simulink model "linearFB"  (R2023a)
settings: Solver=VariableStepAuto  StartTime=0.0  StopTime=60  RelTol=1e-3
values from neighbouring files (symbols this model uses):
  eps_0 = [.2; -.5; .3]    [as5.m]
  eps_c = [-.2; -.4; .2]    [as5.m]
  eta_c = sqrt(1- eps_c'*eps_c)    [as5.m]
  I = [1200 0 0; 0 2000 0; 0 0 2800]    [as5.m]
  k_d = I * eye(3) * 2 * zeta * omega_n    [as5.m]
  k_p = I * eye(3) * 2 * omega_n^2    [as5.m]
  omega_0 = [.1; -.05; .05]    [as5.m]
settings Model: Creator=renob  LastModifiedBy=Josh2

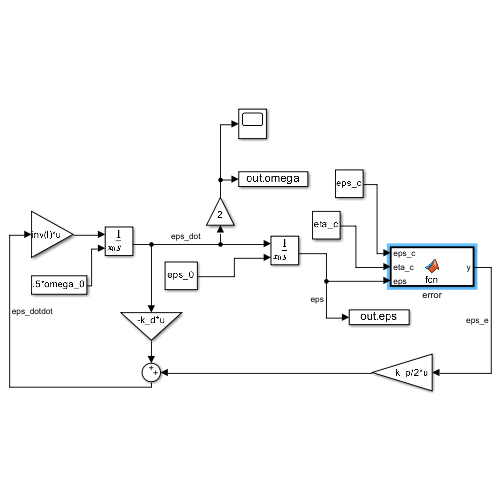
[thumbnail: Simulink's stored preview of the top-level diagram]
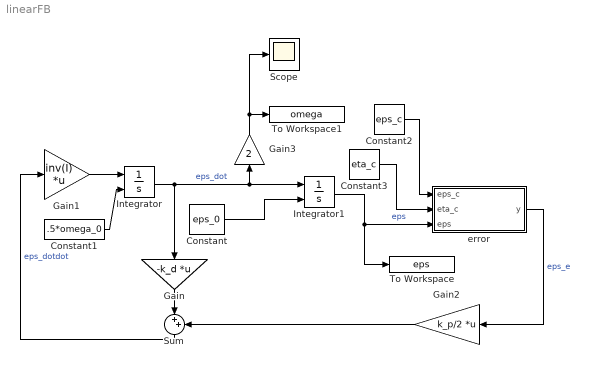
== system linearFB ==
  Constant : Constant  Value=eps_0
  Constant1 : Constant  Value=.5*omega_0
  Constant2 : Constant  Value=eps_c
  Constant3 : Constant  Value=eta_c
  Gain : Gain  Gain=-k_d  Multiplication=Matrix(K*u)
  Gain1 : Gain  Gain=inv(I)  Multiplication=Matrix(K*u)
  Gain2 : Gain  Gain=k_p/2  Multiplication=Matrix(K*u)
  Gain3 : Gain  Gain=2
  Integrator : Integrator  InitialConditionSource=external  InitialCondition=.5*omega_0
  Integrator1 : Integrator  InitialConditionSource=external
  Scope : Scope
  Sum : Sum  Inputs=|++
  To Workspace : ToWorkspace  VariableName=eps  SampleTime=-1
      settings: Save2DSignal=2-D array (concatenate along first dimension)
  To Workspace1 : ToWorkspace  VariableName=omega  SampleTime=-1
      settings: Save2DSignal=2-D array (concatenate along first dimension)
  error : MATLAB Function  TreatAsAtomicUnit=on
  wires:
  Integrator/1 -> Gain/1, Gain3/1, Integrator1/1  "eps_dot"
  Gain1/1 -> Integrator/1
  Integrator1/1 -> To Workspace/1, error/3(eps)  "eps"
  Gain/1 -> Sum/1
  Sum/1 -> Gain1/1  "eps_dotdot"
  Gain2/1 -> Sum/2
  Constant/1 -> Integrator1/2
  Constant1/1 -> Integrator/2
  Gain3/1 -> Scope/1, To Workspace1/1
  error/1(y) -> Gain2/1  "eps_e"
  Constant3/1 -> error/2(eta_c)
  Constant2/1 -> error/1(eps_c)

== matlab function linearFB/error ==
  data: eps_c input; eta_c input; eps input; y output
function y = fcn(eps_c, eta_c, eps)
eta = sqrt(1-eps'*eps);

q_e = quatmultiply(quatconj([eta eps']), [eta_c eps_c']); % assume eta = 1 
y = q_e(2:4)';
